simulink model "Gates"  (R2024b)
settings: Solver=FixedStepAuto  StartTime=0  StopTime=1  FixedStep=0.00001  RelTol=1e-3
libraries: spsTriangleGeneratorLib x1
(part 1 of 2)
settings Model: PacingRate=0.110000  Creator=Erys  LastModifiedBy=Erys

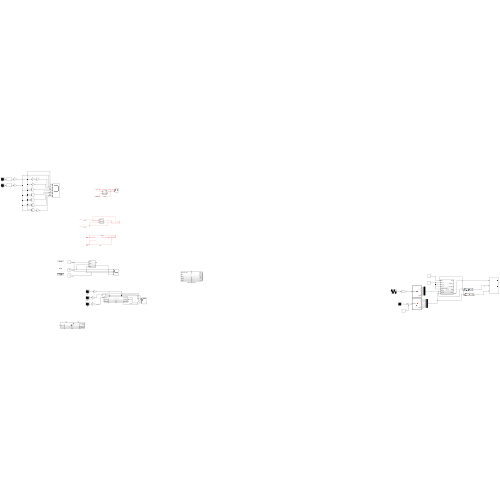
[thumbnail: Simulink's stored preview of the top-level diagram]
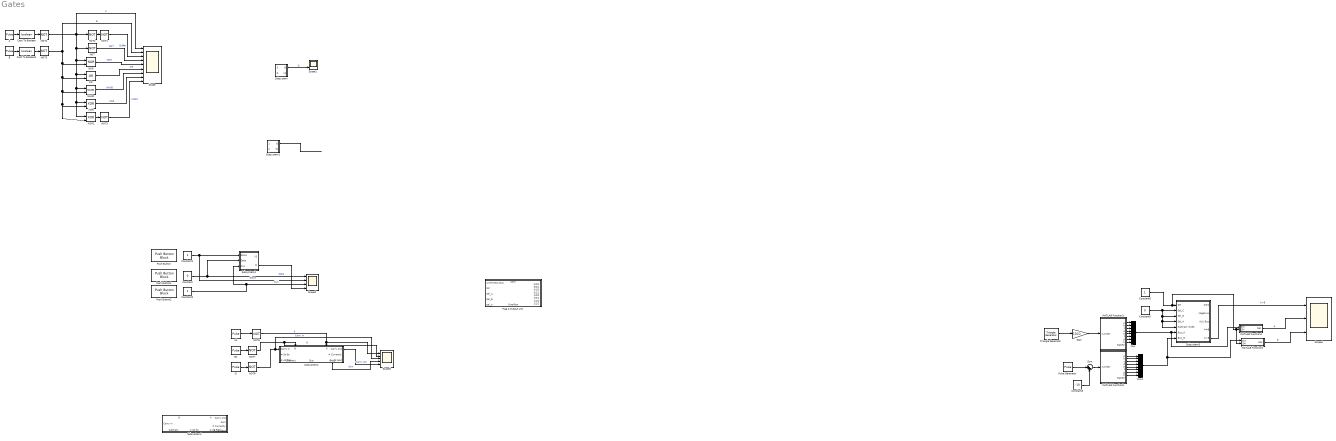
== system Gates ==
  A : DiscretePulseGenerator  PulseType=Time based  Period=1  PulseWidth=50
  A1 : DiscretePulseGenerator  PulseType=Time based  Period=0.25  PulseWidth=50
  B : DiscretePulseGenerator  PulseType=Time based  Period=0.5  PulseWidth=50
  B1 : DiscretePulseGenerator  PulseType=Time based  Period=0.5  PulseWidth=50
  CI : DiscretePulseGenerator  PulseType=Time based  Period=1  PulseWidth=50
  Cast To Boolean : DataTypeConversion  OutDataTypeStr=boolean  SaturateOnIntegerOverflow=off  RndMeth=Floor
  Cast To Boolean1 : DataTypeConversion  OutDataTypeStr=boolean  SaturateOnIntegerOverflow=off  RndMeth=Floor
  Constant : Constant  Value=0  OutDataTypeStr=boolean
  Constant1 : Constant  OutDataTypeStr=boolean
  Constant2 : Constant  OutDataTypeStr=boolean
  Constant3 : Constant  Value=-10
  Constant5 : Constant  Value=0
  Constant6 : Constant
  Flag & Output unit : Subsystem
      settings: PortSchema="{\"entries\":[{\"content\":{\"sides\":[{\"content\":{\"connectorIds\":[\"In1\",\"In2\",\"In3\",\"In4\",\"In5\"]},\"type\":\"ConnectorPlacement.EquallySpacedRectSide\",\"uuid\":\"916d1b19-e284-4a28-84cf-bc055bf0c44e\"},{\"content\":{\"connectorIds\":[\"Out1\",\"Out2\",\"Out3\",\"Out4\",\"Out5\",\"Out6\",\"Out7\",\"Out8\"],\"side\":\"RIGHT\"},\"type\":\"ConnectorPlacement.EquallySpacedRectSide\",\"uuid\":\"7130d779-fd13-4a69-b7b9-2dcd4faf046d\"},{\"content\":{\"connectorIds\":[\"Out9\"],\"side\":\"TOP\"},\"type\":\"ConnectorPlacement.EquallySpacedRectSide\",\"uuid\":\"ce59600e-a31e-4529-9735-bd24f6721c4e\"},{\"content\":{\"connectorIds\":[\"In6\"],\"side\":\"BOTTOM\"},\"type\":\"ConnectorPlacement.EquallySpacedRectSide\",\"uuid\":\"41b3058d-0677-4e1c-be90-f7fc2536099b\"}]},\"type\":\"ConnectorPlacement.EquallySpacedConnector\",\"uuid\":\"b715e1e6-03cb-4b7c-85cc-1984e61b148f\"}],\"packageUris\":[\"http://schema.mathworks.com/mf0/Connector/R2020b\"],\"version\":\"1.0\"}"
  Gain : Gain  Gain=126/2
  MATLAB Function1 : MATLAB Function  TreatAsAtomicUnit=on
  MATLAB Function2 : MATLAB Function  TreatAsAtomicUnit=on
  MATLAB Function3 : MATLAB Function  TreatAsAtomicUnit=on
  MATLAB Function4 : MATLAB Function  TreatAsAtomicUnit=on
  Mux : Mux  Inputs=8
  Mux1 : Mux  Inputs=8
  NAND : Logic  Operator=NAND  IconShape=distinctive  AllPortsSameDT=off  OutDataTypeStr=boolean
  NOR : Logic  Operator=NOR  IconShape=distinctive  AllPortsSameDT=off  OutDataTypeStr=boolean
  NOT{,1..8} (9 alike) : Logic  Operator=NOT  IconShape=distinctive  AllPortsSameDT=off  OutDataTypeStr=boolean
  OR : Logic  Operator=OR  IconShape=distinctive  AllPortsSameDT=off  OutDataTypeStr=boolean
  Pulse Generator : DiscretePulseGenerator  PulseType=Time based  Amplitude=20  Period=1  PulseWidth=50
  Push Button : PushButtonBlock  ButtonType=Latch  OffValue=0.000000
  Push Button1 : PushButtonBlock  ButtonType=Latch  OffValue=0.000000
  Push Button2 : PushButtonBlock  ButtonType=Latch  OffValue=0.000000
  Scope : Scope  NumInputPorts=9
  Scope1 : Scope  NumInputPorts=3
  Scope2 : Scope  NumInputPorts=4
  Scope3 : Scope  NumInputPorts=5
  Scope4 : Scope  NumInputPorts=3
  Subsystem : Subsystem
  Subsystem1 : Subsystem
  Subsystem2 : Subsystem
      settings: PortSchema="{\"entries\":[{\"content\":{\"sides\":[{\"content\":{\"connectorIds\":[\"In1\",\"In2\",\"In3\"]},\"type\":\"ConnectorPlacement.EquallySpacedRectSide\",\"uuid\":\"d566efe6-1fc5-4e96-a6c3-64a47f89d9c9\"},{\"content\":{\"connectorIds\":[\"Out1\",\"Out2\",\"Out3\"],\"side\":\"RIGHT\"},\"type\":\"ConnectorPlacement.EquallySpacedRectSide\",\"uuid\":\"006cd780-973d-4bae-abc8-89f745b28566\"},{\"content\":{\"connectorIds\":[\"In4\",\"In5\"],\"side\":\"TOP\"},\"type\":\"ConnectorPlacement.EquallySpacedRectSide\",\"uuid\":\"c760ecb1-3a5c-4ba0-9224-1c9b5ce710fd\"},{\"content\":{\"connectorIds\":[\"In6\",\"Out4\",\"Out5\"],\"side\":\"BOTTOM\"},\"type\":\"ConnectorPlacement.EquallySpacedRectSide\",\"uuid\":\"178f6c5d-529f-4f0d-80ca-fb6729cf398e\"}]},\"type\":\"ConnectorPlacement.EquallySpacedConnector\",\"uuid\":\"d5293939-72db-46a2-88f3-163e4f70d202\"}],\"packageUris\":[\"http://schema.mathworks.com/mf0/Connector/R2020b\"],\"version\":\"1.0\"}"
  Subsystem3 : Subsystem
  Subsystem4 : Subsystem
      settings: PortSchema="{\"entries\":[{\"content\":{\"sides\":[{\"content\":{\"connectorIds\":[\"In1\"]},\"type\":\"ConnectorPlacement.EquallySpacedRectSide\",\"uuid\":\"d566efe6-1fc5-4e96-a6c3-64a47f89d9c9\"},{\"content\":{\"connectorIds\":[\"Out1\",\"Out2\",\"Out3\",\"Out4\"],\"side\":\"RIGHT\"},\"type\":\"ConnectorPlacement.EquallySpacedRectSide\",\"uuid\":\"006cd780-973d-4bae-abc8-89f745b28566\"},{\"content\":{\"connectorIds\":[\"In2\",\"In3\"],\"side\":\"TOP\"},\"type\":\"ConnectorPlacement.EquallySpacedRectSide\",\"uuid\":\"c760ecb1-3a5c-4ba0-9224-1c9b5ce710fd\"},{\"content\":{\"connectorIds\":[\"In4\",\"In5\",\"In6\"],\"side\":\"BOTTOM\"},\"type\":\"ConnectorPlacement.EquallySpacedRectSide\",\"uuid\":\"178f6c5d-529f-4f0d-80ca-fb6729cf398e\"}]},\"type\":\"ConnectorPlacement.EquallySpacedConnector\",\"uuid\":\"d5293939-72db-46a2-88f3-163e4f70d202\"}],\"packageUris\":[\"http://schema.mathworks.com/mf0/Connector/R2020b\"],\"version\":\"1.0\"}"
  Subsystem5 : Subsystem
  Sum : Sum  Inputs=|++
  Triangle Generator : spsTriangleGeneratorLib/Triangle Generator  Freq=4  Phase=90  Ts=0
  XOR : Logic  Operator=XOR  IconShape=distinctive  AllPortsSameDT=off  OutDataTypeStr=boolean
  XOR1 : Logic  Operator=XOR  IconShape=distinctive  AllPortsSameDT=off  OutDataTypeStr=boolean
  wires:
  NOT2/1 -> NOT1/1
  XOR1/1 -> NOT3/1
  A/1 -> Cast To Boolean/1
  B/1 -> Cast To Boolean1/1
  NOR/1 -> Scope/5  "NOR"
  Cast To Boolean/1 -> NOT4/1
  Cast To Boolean1/1 -> NOT5/1
  NOT4/1 -> XOR1/1, XOR/1, NAND/1, OR/1, NOR/1, NOT/1, Scope/1, NOT2/1  "A"
  NOT5/1 -> XOR1/2, XOR/2, NAND/2, OR/2, NOR/2, Scope/2  "B"
  NOT1/1 -> Scope/3  "Buffer"
  NOT/1 -> Scope/4  "NOT"
  OR/1 -> Scope/6  "OR"
  NAND/1 -> Scope/7  "NAND"
  XOR/1 -> Scope/8  "XOR"
  NOT3/1 -> Scope/9  "XNOR"
  ? -> Scope1/2, Subsystem/2(R)  "Reset"
  ? -> Scope1/1, Subsystem/1(S)  "Set"
  Subsystem/1(Q) -> Scope1/3  "Q"
  ? -> Subsystem1/1(Data)  "Data"
  ? -> Subsystem1/2(CLK)  "CLK"
  Subsystem1/1(Q) -> ?
  ? -> ?  "Data"
  ? -> ?  "CLK"
  ? -> ?  "Q"
  Constant1/1 -> Scope2/2, Subsystem3/1(Store)  "Store"
  Constant/1 -> Scope2/1, Subsystem3/2(Data)  "Data"
  Constant2/1 -> Subsystem3/3(CLK), Scope2/3  "CLK"
  Subsystem3/2(Q) -> Scope2/4
  A1/1 -> NOT6/1
  B1/1 -> NOT7/1
  CI/1 -> NOT8/1
  Subsystem2/5(Out1) -> Scope3/4  "Sum"
  Subsystem2/1(Carry Out) -> Scope3/5  "Carry out"
  NOT6/1 -> Scope3/1, Subsystem2/5(A)  "A"
  NOT7/1 -> Scope3/2, Subsystem2/4(B)  "B"
  NOT8/1 -> Scope3/3, Subsystem2/1(Carry In)  "Carry In"
  MATLAB Function1/8(h) -> Mux/8
  MATLAB Function1/4(d) -> Mux/4
  MATLAB Function1/7(g) -> Mux/7
  MATLAB Function1/6(f) -> Mux/6
  MATLAB Function1/3(c) -> Mux/3
  MATLAB Function1/1(a) -> Mux/1
  MATLAB Function1/5(e) -> Mux/5
  MATLAB Function1/2(b) -> Mux/2
  Constant5/1 -> Subsystem5/5(Subtract mode), Subsystem5/4(Sel_A), Subsystem5/3(Sel_B), Subsystem5/2(Sel_C)
  MATLAB Function3/5(e) -> Mux1/5
  MATLAB Function3/1(a) -> Mux1/1
  MATLAB Function3/2(b) -> Mux1/2
  Mux1/1 -> MATLAB Function2/1(Bin), Subsystem5/7(Bus_B)
  MATLAB Function3/4(d) -> Mux1/4
  MATLAB Function3/7(g) -> Mux1/7
  MATLAB Function3/8(h) -> Mux1/8
  MATLAB Function3/3(c) -> Mux1/3
  MATLAB Function3/6(f) -> Mux1/6
  Mux/1 -> MATLAB Function4/1(Bin), Subsystem5/6(Bus_A)
  MATLAB Function4/1(Dec) -> Scope4/2  "A"
  MATLAB Function2/1(Dec) -> Scope4/3  "B"
  Constant6/1 -> MATLAB Function2/2(SM), MATLAB Function4/2(SM), Subsystem5/1(SM)
  Subsystem5/5(A>B) -> Scope4/1  "A>B"
  Gain/1 -> MATLAB Function1/1(number)
  Triangle Generator/1 -> Gain/1
  Pulse Generator/1 -> Sum/1
  Sum/1 -> MATLAB Function3/1(number)
  Constant3/1 -> Sum/2

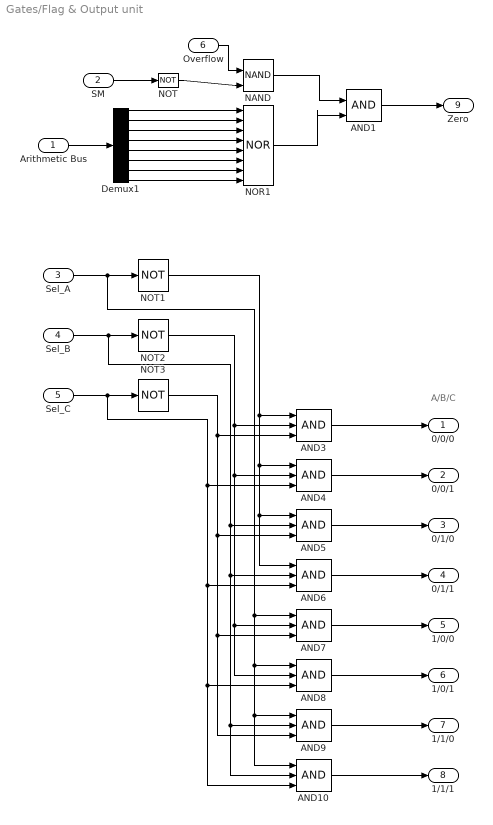
== system Gates/Flag & Output unit ==
  note: A/B/C
  Arithmetic Bus : Inport
  SM : Inport  Port=2
  Sel_A : Inport  Port=3
  Sel_B : Inport  Port=4
  Sel_C : Inport  Port=5
  Overflow : Inport  Port=6
  AND1 : Logic  IconShape=distinctive  AllPortsSameDT=off  OutDataTypeStr=boolean
  AND{3..10} (8 alike) : Logic  Inputs=3  IconShape=distinctive  AllPortsSameDT=off  OutDataTypeStr=boolean
  Demux1 : Demux  Outputs=8
  NAND : Logic  Operator=NAND  IconShape=distinctive  AllPortsSameDT=off  OutDataTypeStr=boolean
  NOR1 : Logic  Operator=NOR  Inputs=8  IconShape=distinctive  AllPortsSameDT=off  OutDataTypeStr=boolean
  NOT{,1..3} (4 alike) : Logic  Operator=NOT  IconShape=distinctive  AllPortsSameDT=off  OutDataTypeStr=boolean
  0/0/0 : Outport
  0/0/1 : Outport  Port=2
  0/1/0 : Outport  Port=3
  0/1/1 : Outport  Port=4
  1/0/0 : Outport  Port=5
  1/0/1 : Outport  Port=6
  1/1/0 : Outport  Port=7
  1/1/1 : Outport  Port=8
  Zero : Outport  Port=9
  wires:
  SM/1 -> NOT/1
  Demux1/1 -> NOR1/1
  NOT/1 -> NAND/2
  Demux1/4 -> NOR1/4
  NOR1/1 -> AND1/2
  Overflow/1 -> NAND/1
  Demux1/5 -> NOR1/5
  NAND/1 -> AND1/1
  Demux1/8 -> NOR1/8
  Demux1/6 -> NOR1/6
  Arithmetic Bus/1 -> Demux1/1
  Demux1/7 -> NOR1/7
  Demux1/3 -> NOR1/3
  AND1/1 -> Zero/1
  Demux1/2 -> NOR1/2
  AND3/1 -> 0/0/0/1
  NOT1/1 -> AND6/1, AND5/1, AND4/1, AND3/1
  AND9/1 -> 1/1/0/1
  Sel_C/1 -> AND10/3, AND8/3, AND6/3, AND4/3, NOT3/1
  AND7/1 -> 1/0/0/1
  AND6/1 -> 0/1/1/1
  NOT2/1 -> AND4/2, AND7/2, AND8/2, AND3/2
  Sel_B/1 -> AND10/2, AND9/2, AND6/2, AND5/2, NOT2/1
  AND4/1 -> 0/0/1/1
  NOT3/1 -> AND9/3, AND7/3, AND5/3, AND3/3
  Sel_A/1 -> AND10/1, AND9/1, AND8/1, AND7/1, NOT1/1
  AND5/1 -> 0/1/0/1
  AND8/1 -> 1/0/1/1
  AND10/1 -> 1/1/1/1

== system Gates/Subsystem ==
  S : Inport
  R : Inport  Port=2
  Delay One Step : Delay  DelayLength=1
  NOR1 : Logic  Operator=NOR  IconShape=distinctive  AllPortsSameDT=off  OutDataTypeStr=boolean
  NOR2 : Logic  Operator=NOR  IconShape=distinctive  AllPortsSameDT=off  OutDataTypeStr=boolean
  Q : Outport
  !Q : Outport  Port=2
  wires:
  Delay One Step/1 -> NOR1/2, Q/1  "Q"
  S/1 -> NOR1/1
  R/1 -> NOR2/2
  NOR1/1 -> !Q/1, NOR2/1
  NOR2/1 -> Delay One Step/1

== system Gates/Subsystem1 ==
  Data : Inport
  CLK : Inport  Port=2
  Delay One Step : Delay  DelayLength=1
  NAND{1..4} (4 alike) : Logic  Operator=NAND  IconShape=distinctive  AllPortsSameDT=off  OutDataTypeStr=boolean
  Q : Outport
  !Q : Outport  Port=2
  wires:
  NAND1/1 -> Delay One Step/1
  NAND4/1 -> NAND2/2
  Delay One Step/1 -> NAND2/1, Q/1  "Q"
  NAND2/1 -> !Q/1, NAND1/2
  NAND3/1 -> NAND4/1, NAND1/1
  CLK/1 -> NAND3/2, NAND4/2
  Data/1 -> NAND3/1

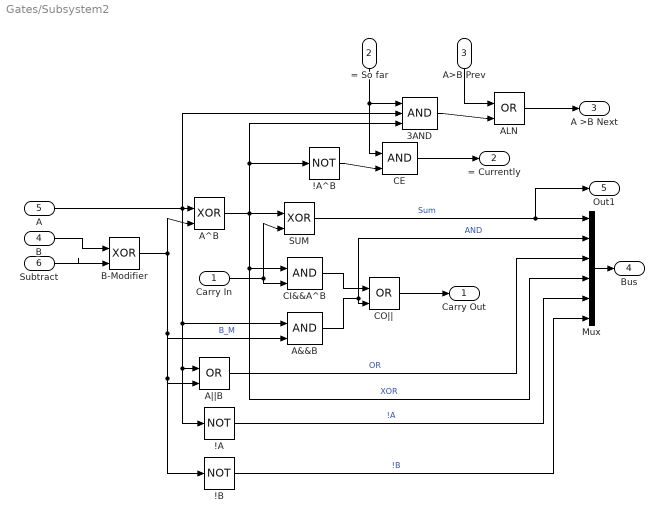
== system Gates/Subsystem2 ==
  Carry In : Inport
  = So far : Inport  Port=2
  A>B Prev : Inport  Port=3
  B : Inport  Port=4
  A : Inport  Port=5
  Subtract : Inport  Port=6
  !A : Logic  Operator=NOT  IconShape=distinctive  AllPortsSameDT=off  OutDataTypeStr=boolean
  !A^B : Logic  Operator=NOT  IconShape=distinctive  AllPortsSameDT=off  OutDataTypeStr=boolean
  !B : Logic  Operator=NOT  IconShape=distinctive  AllPortsSameDT=off  OutDataTypeStr=boolean
  3AND : Logic  Inputs=3  IconShape=distinctive  AllPortsSameDT=off  OutDataTypeStr=boolean
  A&&B : Logic  IconShape=distinctive  AllPortsSameDT=off  OutDataTypeStr=boolean
  ALN : Logic  Operator=OR  IconShape=distinctive  AllPortsSameDT=off  OutDataTypeStr=boolean
  A^B : Logic  Operator=XOR  IconShape=distinctive  AllPortsSameDT=off  OutDataTypeStr=boolean
  A||B : Logic  Operator=OR  IconShape=distinctive  AllPortsSameDT=off  OutDataTypeStr=boolean
  B-Modifier : Logic  Operator=XOR  IconShape=distinctive  AllPortsSameDT=off  OutDataTypeStr=boolean
  CE : Logic  IconShape=distinctive  AllPortsSameDT=off  OutDataTypeStr=boolean
  CI&&A^B : Logic  IconShape=distinctive  AllPortsSameDT=off  OutDataTypeStr=boolean
  CO|| : Logic  Operator=OR  IconShape=distinctive  AllPortsSameDT=off  OutDataTypeStr=boolean
  Mux : Mux  Inputs=6
  SUM : Logic  Operator=XOR  IconShape=distinctive  AllPortsSameDT=off  OutDataTypeStr=boolean
  Carry Out : Outport
  = Currently : Outport  Port=2
  A >B Next : Outport  Port=3
  Bus : Outport  Port=4
  Out1 : Outport  Port=5
  wires:
  B/1 -> B-Modifier/1
  Subtract/1 -> B-Modifier/2
  CI&&A^B/1 -> CO||/1
  A&&B/1 -> Mux/2, CO||/2  "AND"
  CO||/1 -> Carry Out/1
  B-Modifier/1 -> A&&B/2, !B/1, A||B/2, A^B/2  "B_M"
  Carry In/1 -> CI&&A^B/2, SUM/2
  SUM/1 -> Out1/1, Mux/1  "Sum"
  A^B/1 -> Mux/4, CI&&A^B/1, 3AND/3, !A^B/1, SUM/1  "XOR"
  A>B Prev/1 -> ALN/1
  ALN/1 -> A >B Next/1
  !A^B/1 -> CE/2
  CE/1 -> = Currently/1
  3AND/1 -> ALN/2
  A/1 -> !A/1, A||B/1, A&&B/1, A^B/1, 3AND/2
  = So far/1 -> CE/1, 3AND/1
  A||B/1 -> Mux/3  "OR"
  Mux/1 -> Bus/1
  !A/1 -> Mux/5  "!A"
  !B/1 -> Mux/6  "!B"

== system Gates/Subsystem3 ==
  Store : Inport
  Data : Inport  Port=2
  CLK : Inport  Port=3
  NAND1 : Logic  Operator=NAND  IconShape=distinctive  AllPortsSameDT=off  OutDataTypeStr=boolean
  NAND2 : Logic  Operator=NAND  IconShape=distinctive  AllPortsSameDT=off  OutDataTypeStr=boolean
  NAND3 : Logic  Operator=NAND  IconShape=distinctive  AllPortsSameDT=off  OutDataTypeStr=boolean
  NOT6 : Logic  Operator=NOT  IconShape=distinctive  AllPortsSameDT=off  OutDataTypeStr=boolean
  Subsystem2 : Subsystem
  !Q : Outport
  Q : Outport  Port=2
  wires:
  NAND3/1 -> NAND1/2
  Subsystem2/1(Q) -> Q/1, NAND2/1  "Q"
  NAND1/1 -> Subsystem2/1(Data)
  NOT6/1 -> NAND2/2
  CLK/1 -> Subsystem2/2(CLK)
  Store/1 -> NOT6/1, NAND3/1
  NAND2/1 -> NAND1/1
  Subsystem2/2(!Q) -> !Q/1
  Data/1 -> NAND3/2

== system Gates/Subsystem4 ==
  Carry In : Inport
  B : Inport  Port=2
  A : Inport  Port=3
  Subtract : Inport  Port=4
  = So far : Inport  Port=5
  A>B Prev : Inport  Port=6
  !A^B : Logic  Operator=NOT  IconShape=distinctive  AllPortsSameDT=off  OutDataTypeStr=boolean
  AND : Logic  IconShape=distinctive  AllPortsSameDT=off  OutDataTypeStr=boolean
  AND2 : Logic  IconShape=distinctive  AllPortsSameDT=off  OutDataTypeStr=boolean
  AND5 : Logic  IconShape=distinctive  AllPortsSameDT=off  OutDataTypeStr=boolean
  AND6 : Logic  Inputs=3  IconShape=distinctive  AllPortsSameDT=off  OutDataTypeStr=boolean
  OR1 : Logic  Operator=OR  IconShape=distinctive  AllPortsSameDT=off  OutDataTypeStr=boolean
  OR2 : Logic  Operator=OR  IconShape=distinctive  AllPortsSameDT=off  OutDataTypeStr=boolean
  XOR : Logic  Operator=XOR  IconShape=distinctive  AllPortsSameDT=off  OutDataTypeStr=boolean
  XOR1 : Logic  Operator=XOR  IconShape=distinctive  AllPortsSameDT=off  OutDataTypeStr=boolean
  XOR2 : Logic  Operator=XOR  IconShape=distinctive  AllPortsSameDT=off  OutDataTypeStr=boolean
  Carry Out : Outport
  Sum : Outport  Port=2
  = Currently : Outport  Port=3
  A >B Next : Outport  Port=4
  wires:
  B/1 -> XOR1/1
  Subtract/1 -> XOR1/2
  AND/1 -> OR1/1
  AND2/1 -> OR1/2
  OR1/1 -> Carry Out/1
  XOR1/1 -> AND2/2, XOR2/2
  Carry In/1 -> AND/2, XOR/2
  XOR/1 -> Sum/1
  AND5/1 -> = Currently/1
  = So far/1 -> AND6/1, AND5/1
  !A^B/1 -> AND5/2
  XOR2/1 -> AND6/3, !A^B/1, AND/1, XOR/1
  OR2/1 -> A >B Next/1
  A/1 -> AND2/1, AND6/2, XOR2/1
  AND6/1 -> OR2/2
  A>B Prev/1 -> OR2/1

== system Gates/Subsystem5 ==
  SM : Inport
  Sel_C : Inport  Port=2
  Sel_B : Inport  Port=3
  Sel_A : Inport  Port=4
  Subtract mode : Inport  Port=5
  Bus_A : Inport  Port=6
  Bus_B : Inport  Port=7
  ALU Selector Bus : Subsystem
      settings: PortSchema="{\"entries\":[{\"content\":{\"sides\":[{\"content\":{\"connectorIds\":[\"In1\",\"In2\",\"In3\",\"In4\",\"In5\",\"In6\",\"In7\",\"In8\",\"In9\",\"In10\",\"In11\",\"In12\",\"In13\",\"In14\",\"In15\",\"In16\"]},\"type\":\"ConnectorPlacement.EquallySpacedRectSide\",\"uuid\":\"e3413fa4-1b2d-4ebe-83ea-8face2a722c4\"},{\"content\":{\"side\":\"RIGHT\"},\"type\":\"ConnectorPlacement.EquallySpacedRectSide\",\"uuid\":\"468a20b8-3e48-40d2-af84-5907293b05d2\"},{\"content\":{\"connectorIds\":[\"Out1\"],\"side\":\"TOP\"},\"type\":\"ConnectorPlacement.EquallySpacedRectSide\",\"uuid\":\"4c8356f8-7f0f-47fd-8d6e-25cf38d6ddc3\"}]},\"type\":\"ConnectorPlacement.EquallySpacedConnector\",\"uuid\":\"84f87871-f62c-4317-8781-2bab8d5e1233\"}],\"packageUris\":[\"http://schema.mathworks.com/mf0/Connector/R2020b\"],\"version\":\"1.0\"}"
  Adder & Logic Module : Subsystem
      settings: PortSchema="{\"entries\":[{\"content\":{\"sides\":[{\"content\":{\"connectorIds\":[\"In1\",\"In2\"]},\"type\":\"ConnectorPlacement.EquallySpacedRectSide\",\"uuid\":\"639aed8e-35a1-4ba0-8b43-3214fbb2c368\"},{\"content\":{\"connectorIds\":[\"Out1\",\"Out2\",\"Out3\",\"Out4\",\"Out5\",\"Out6\",\"Out7\",\"Out8\"],\"side\":\"RIGHT\"},\"type\":\"ConnectorPlacement.EquallySpacedRectSide\",\"uuid\":\"8a439bfb-ce30-47da-a5b4-a54b9d9e640c\"},{\"content\":{\"connectorIds\":[\"In3\",\"Out11\"],\"side\":\"TOP\"},\"type\":\"ConnectorPlacement.EquallySpacedRectSide\",\"uuid\":\"7d81641d-429b-4b81-8cb3-af5c318085c9\"},{\"content\":{\"connectorIds\":[\"Out9\",\"Out10\"],\"side\":\"BOTTOM\"},\"type\":\"ConnectorPlacement.EquallySpacedRectSide\",\"uuid\":\"74152c7b-6851-457b-b5de-2c09c1f82f74\"}]},\"type\":\"ConnectorPlacement.EquallySpacedConnector\",\"uuid\":\"d9b5c2cc-0f19-487b-a2d0-c7259543056d\"}],\"packageUris\":[\"http://schema.mathworks.com/mf0/Connector/R2020b\"],\"version\":\"1.0\"}"
  Flag & Output unit1 : Subsystem
      settings: PortSchema="{\"entries\":[{\"content\":{\"sides\":[{\"content\":{\"connectorIds\":[\"In1\",\"In2\",\"In3\",\"In4\"]},\"type\":\"ConnectorPlacement.EquallySpacedRectSide\",\"uuid\":\"916d1b19-e284-4a28-84cf-bc055bf0c44e\"},{\"content\":{\"connectorIds\":[\"Out1\",\"Out2\",\"Out3\",\"Out4\",\"Out5\",\"Out6\",\"Out7\",\"Out8\"],\"side\":\"RIGHT\"},\"type\":\"ConnectorPlacement.EquallySpacedRectSide\",\"uuid\":\"7130d779-fd13-4a69-b7b9-2dcd4faf046d\"},{\"content\":{\"connectorIds\":[\"Out9\",\"Out10\",\"In5\"],\"side\":\"TOP\"},\"type\":\"ConnectorPlacement.EquallySpacedRectSide\",\"uuid\":\"ce59600e-a31e-4529-9735-bd24f6721c4e\"},{\"content\":{\"connectorIds\":[\"In6\"],\"side\":\"BOTTOM\"},\"type\":\"ConnectorPlacement.EquallySpacedRectSide\",\"uuid\":\"41b3058d-0677-4e1c-be90-f7fc2536099b\"}]},\"type\":\"ConnectorPlacement.EquallySpacedConnector\",\"uuid\":\"b715e1e6-03cb-4b7c-85cc-1984e61b148f\"}],\"packageUris\":[\"http://schema.mathworks.com/mf0/Connector/R2020b\"],\"version\":\"1.0\"}"
  Zero : Outport
  Negative : Outport  Port=2
  ALU Bus : Outport  Port=3
  A=B : Outport  Port=4
  A>B : Outport  Port=5
  wires:
  Subtract mode/1 -> Adder & Logic Module/3(Subtract mode)
  Bus_B/1 -> Adder & Logic Module/2(Bus_B)
  Bus_A/1 -> Adder & Logic Module/1(Bus_A)
  Adder & Logic Module/10(A>B) -> A>B/1
  Adder & Logic Module/7(Bus7) -> ALU Selector Bus/15(Bus7)
  Adder & Logic Module/5(Bus5) -> ALU Selector Bus/13(Bus5)
  Adder & Logic Module/3(Bus3) -> ALU Selector Bus/11(Bus3)
  Adder & Logic Module/9(A=B) -> A=B/1
  SM/1 -> Flag & Output unit1/1(SM)
  Sel_B/1 -> Flag & Output unit1/3(Sel_B)
  Sel_A/1 -> Flag & Output unit1/2(Sel_A)
  Sel_C/1 -> Flag & Output unit1/4(Sel_C)
  Adder & Logic Module/1(Bus1) -> ALU Selector Bus/9(Bus1)
  Adder & Logic Module/8(Bus8) -> ALU Selector Bus/16(Bus8)
  Adder & Logic Module/6(Bus6) -> ALU Selector Bus/14(Bus6)
  Adder & Logic Module/4(Bus4) -> ALU Selector Bus/12(Bus4)
  Adder & Logic Module/2(Bus2) -> ALU Selector Bus/10(Bus2)
  Adder & Logic Module/11(Overflow) -> Flag & Output unit1/6(Overflow)
  Flag & Output unit1/5(1/0/0) -> ALU Selector Bus/5(1/0/0)
  Flag & Output unit1/3(0/1/0) -> ALU Selector Bus/3(0/1/0)
  Flag & Output unit1/1(0/0/0) -> ALU Selector Bus/1(0/0/0)
  Flag & Output unit1/4(0/1/1) -> ALU Selector Bus/4(0/1/1)
  Flag & Output unit1/2(0/0/1) -> ALU Selector Bus/2(0/0/1)
  Flag & Output unit1/10(Negative) -> Negative/1
  Flag & Output unit1/8(1/1/1) -> ALU Selector Bus/8(1/1/1)
  Flag & Output unit1/6(1/0/1) -> ALU Selector Bus/6(1/0/1)
  Flag & Output unit1/9(Zero) -> Zero/1
  Flag & Output unit1/7(1/1/0) -> ALU Selector Bus/7(1/1/0)
  ALU Selector Bus/1(ALU Output) -> Flag & Output unit1/5(ALU Bus), ALU Bus/1

== system Gates/Subsystem3/Subsystem2 ==
  Data : Inport
  CLK : Inport  Port=2
  DLatch Master : Subsystem
  DLatch Slave : Subsystem
  NOT6 : Logic  Operator=NOT  IconShape=distinctive  AllPortsSameDT=off  OutDataTypeStr=boolean
  Q : Outport
  !Q : Outport  Port=2
  wires:
  DLatch Master/1(Q) -> DLatch Slave/1(Data)
  NOT6/1 -> DLatch Master/2(CLK)
  CLK/1 -> DLatch Slave/2(CLK), NOT6/1
  Data/1 -> DLatch Master/1(Data)
  DLatch Slave/1(Q) -> Q/1
  DLatch Slave/2(!Q) -> !Q/1

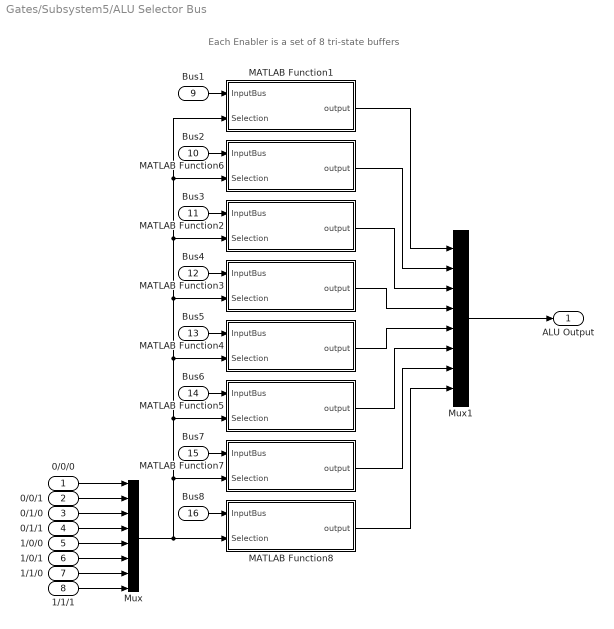
== system Gates/Subsystem5/ALU Selector Bus ==
  note: Each Enabler is a set of 8 tri-state buffers
  0/0/0 : Inport
  0/0/1 : Inport  Port=2
  0/1/0 : Inport  Port=3
  0/1/1 : Inport  Port=4
  1/0/0 : Inport  Port=5
  1/0/1 : Inport  Port=6
  1/1/0 : Inport  Port=7
  1/1/1 : Inport  Port=8
  Bus1 : Inport  Port=9
  Bus2 : Inport  Port=10
  Bus3 : Inport  Port=11
  Bus4 : Inport  Port=12
  Bus5 : Inport  Port=13
  Bus6 : Inport  Port=14
  Bus7 : Inport  Port=15
  Bus8 : Inport  Port=16
  MATLAB Function1 : MATLAB Function  TreatAsAtomicUnit=on
  MATLAB Function2 : MATLAB Function  TreatAsAtomicUnit=on
  MATLAB Function3 : MATLAB Function  TreatAsAtomicUnit=on
  MATLAB Function4 : MATLAB Function  TreatAsAtomicUnit=on
  MATLAB Function5 : MATLAB Function  TreatAsAtomicUnit=on
  MATLAB Function6 : MATLAB Function  TreatAsAtomicUnit=on
  MATLAB Function7 : MATLAB Function  TreatAsAtomicUnit=on
  MATLAB Function8 : MATLAB Function  TreatAsAtomicUnit=on
  Mux : Mux  Inputs=8
  Mux1 : Mux  Inputs=8
  ALU Output : Outport
  wires:
  1/1/1/1 -> Mux/8
  1/1/0/1 -> Mux/7
  1/0/1/1 -> Mux/6
  1/0/0/1 -> Mux/5
  0/1/1/1 -> Mux/4
  0/1/0/1 -> Mux/3
  0/0/1/1 -> Mux/2
  0/0/0/1 -> Mux/1
  Bus3/1 -> MATLAB Function2/1(InputBus)
  Bus5/1 -> MATLAB Function4/1(InputBus)
  Bus8/1 -> MATLAB Function8/1(InputBus)
  Bus2/1 -> MATLAB Function6/1(InputBus)
  Bus4/1 -> MATLAB Function3/1(InputBus)
  Bus1/1 -> MATLAB Function1/1(InputBus)
  Bus6/1 -> MATLAB Function5/1(InputBus)
  Bus7/1 -> MATLAB Function7/1(InputBus)
  Mux/1 -> MATLAB Function8/2(Selection), MATLAB Function7/2(Selection), MATLAB Function5/2(Selection), MATLAB Function4/2(Selection), MATLAB Function3/2(Selection), MATLAB Function2/2(Selection), MATLAB Function1/2(Selection), MATLAB Function6/2(Selection)
  MATLAB Function6/1(output) -> Mux1/2
  MATLAB Function2/1(output) -> Mux1/3
  MATLAB Function3/1(output) -> Mux1/4
  MATLAB Function4/1(output) -> Mux1/5
  MATLAB Function5/1(output) -> Mux1/6
  MATLAB Function7/1(output) -> Mux1/7
  MATLAB Function8/1(output) -> Mux1/8
  MATLAB Function1/1(output) -> Mux1/1
  Mux1/1 -> ALU Output/1

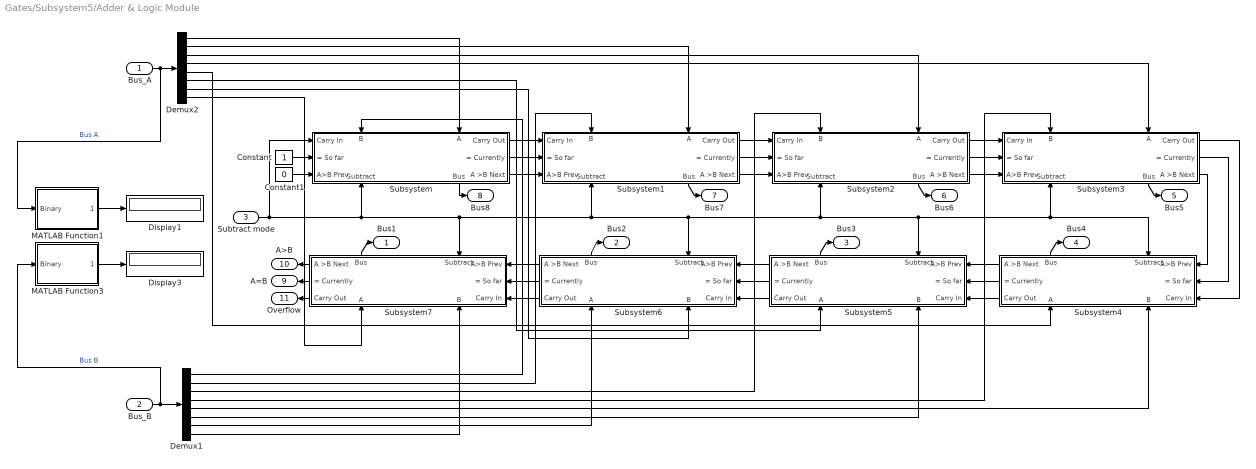
== system Gates/Subsystem5/Adder & Logic Module ==
  Bus_A : Inport
  Bus_B : Inport  Port=2
  Subtract mode : Inport  Port=3
  Constant : Constant
  Constant1 : Constant  Value=0
  Demux1 : Demux  Outputs=8
  Demux2 : Demux  Outputs=8
  Display1 : Display
  Display3 : Display
  MATLAB Function1 : MATLAB Function  TreatAsAtomicUnit=on
  MATLAB Function3 : MATLAB Function  TreatAsAtomicUnit=on
  Subsystem : Subsystem
      settings: PortSchema="{\"entries\":[{\"content\":{\"sides\":[{\"content\":{\"connectorIds\":[\"In1\",\"In2\",\"In3\"]},\"type\":\"ConnectorPlacement.EquallySpacedRectSide\",\"uuid\":\"d566efe6-1fc5-4e96-a6c3-64a47f89d9c9\"},{\"content\":{\"connectorIds\":[\"Out1\",\"Out2\",\"Out3\"],\"side\":\"RIGHT\"},\"type\":\"ConnectorPlacement.EquallySpacedRectSide\",\"uuid\":\"006cd780-973d-4bae-abc8-89f745b28566\"},{\"content\":{\"connectorIds\":[\"In4\",\"In5\"],\"side\":\"TOP\"},\"type\":\"ConnectorPlacement.EquallySpacedRectSide\",\"uuid\":\"c760ecb1-3a5c-4ba0-9224-1c9b5ce710fd\"},{\"content\":{\"connectorIds\":[\"In6\",\"Out4\"],\"side\":\"BOTTOM\"},\"type\":\"ConnectorPlacement.EquallySpacedRectSide\",\"uuid\":\"178f6c5d-529f-4f0d-80ca-fb6729cf398e\"}]},\"type\":\"ConnectorPlacement.EquallySpacedConnector\",\"uuid\":\"d5293939-72db-46a2-88f3-163e4f70d202\"}],\"packageUris\":[\"http://schema.mathworks.com/mf0/Connector/R2020b\"],\"version\":\"1.0\"}"
  Subsystem1 : Subsystem
      settings: PortSchema="{\"entries\":[{\"content\":{\"sides\":[{\"content\":{\"connectorIds\":[\"In1\",\"In2\",\"In3\"]},\"type\":\"ConnectorPlacement.EquallySpacedRectSide\",\"uuid\":\"d566efe6-1fc5-4e96-a6c3-64a47f89d9c9\"},{\"content\":{\"connectorIds\":[\"Out1\",\"Out2\",\"Out3\"],\"side\":\"RIGHT\"},\"type\":\"ConnectorPlacement.EquallySpacedRectSide\",\"uuid\":\"006cd780-973d-4bae-abc8-89f745b28566\"},{\"content\":{\"connectorIds\":[\"In4\",\"In5\"],\"side\":\"TOP\"},\"type\":\"ConnectorPlacement.EquallySpacedRectSide\",\"uuid\":\"c760ecb1-3a5c-4ba0-9224-1c9b5ce710fd\"},{\"content\":{\"connectorIds\":[\"In6\",\"Out4\"],\"side\":\"BOTTOM\"},\"type\":\"ConnectorPlacement.EquallySpacedRectSide\",\"uuid\":\"178f6c5d-529f-4f0d-80ca-fb6729cf398e\"}]},\"type\":\"ConnectorPlacement.EquallySpacedConnector\",\"uuid\":\"d5293939-72db-46a2-88f3-163e4f70d202\"}],\"packageUris\":[\"http://schema.mathworks.com/mf0/Connector/R2020b\"],\"version\":\"1.0\"}"
  Subsystem2 : Subsystem
      settings: PortSchema="{\"entries\":[{\"content\":{\"sides\":[{\"content\":{\"connectorIds\":[\"In1\",\"In2\",\"In3\"]},\"type\":\"ConnectorPlacement.EquallySpacedRectSide\",\"uuid\":\"d566efe6-1fc5-4e96-a6c3-64a47f89d9c9\"},{\"content\":{\"connectorIds\":[\"Out1\",\"Out2\",\"Out3\"],\"side\":\"RIGHT\"},\"type\":\"ConnectorPlacement.EquallySpacedRectSide\",\"uuid\":\"006cd780-973d-4bae-abc8-89f745b28566\"},{\"content\":{\"connectorIds\":[\"In4\",\"In5\"],\"side\":\"TOP\"},\"type\":\"ConnectorPlacement.EquallySpacedRectSide\",\"uuid\":\"c760ecb1-3a5c-4ba0-9224-1c9b5ce710fd\"},{\"content\":{\"connectorIds\":[\"In6\",\"Out4\"],\"side\":\"BOTTOM\"},\"type\":\"ConnectorPlacement.EquallySpacedRectSide\",\"uuid\":\"178f6c5d-529f-4f0d-80ca-fb6729cf398e\"}]},\"type\":\"ConnectorPlacement.EquallySpacedConnector\",\"uuid\":\"d5293939-72db-46a2-88f3-163e4f70d202\"}],\"packageUris\":[\"http://schema.mathworks.com/mf0/Connector/R2020b\"],\"version\":\"1.0\"}"
  Subsystem3 : Subsystem
      settings: PortSchema="{\"entries\":[{\"content\":{\"sides\":[{\"content\":{\"connectorIds\":[\"In1\",\"In2\",\"In3\"]},\"type\":\"ConnectorPlacement.EquallySpacedRectSide\",\"uuid\":\"d566efe6-1fc5-4e96-a6c3-64a47f89d9c9\"},{\"content\":{\"connectorIds\":[\"Out1\",\"Out2\",\"Out3\"],\"side\":\"RIGHT\"},\"type\":\"ConnectorPlacement.EquallySpacedRectSide\",\"uuid\":\"006cd780-973d-4bae-abc8-89f745b28566\"},{\"content\":{\"connectorIds\":[\"In4\",\"In5\"],\"side\":\"TOP\"},\"type\":\"ConnectorPlacement.EquallySpacedRectSide\",\"uuid\":\"c760ecb1-3a5c-4ba0-9224-1c9b5ce710fd\"},{\"content\":{\"connectorIds\":[\"In6\",\"Out4\"],\"side\":\"BOTTOM\"},\"type\":\"ConnectorPlacement.EquallySpacedRectSide\",\"uuid\":\"178f6c5d-529f-4f0d-80ca-fb6729cf398e\"}]},\"type\":\"ConnectorPlacement.EquallySpacedConnector\",\"uuid\":\"d5293939-72db-46a2-88f3-163e4f70d202\"}],\"packageUris\":[\"http://schema.mathworks.com/mf0/Connector/R2020b\"],\"version\":\"1.0\"}"
  Subsystem4 : Subsystem
      settings: PortSchema="{\"entries\":[{\"content\":{\"sides\":[{\"content\":{\"connectorIds\":[\"In1\",\"In2\",\"In3\"]},\"type\":\"ConnectorPlacement.EquallySpacedRectSide\",\"uuid\":\"d566efe6-1fc5-4e96-a6c3-64a47f89d9c9\"},{\"content\":{\"connectorIds\":[\"Out1\",\"Out2\",\"Out3\"],\"side\":\"RIGHT\"},\"type\":\"ConnectorPlacement.EquallySpacedRectSide\",\"uuid\":\"006cd780-973d-4bae-abc8-89f745b28566\"},{\"content\":{\"connectorIds\":[\"In4\",\"In5\"],\"side\":\"TOP\"},\"type\":\"ConnectorPlacement.EquallySpacedRectSide\",\"uuid\":\"c760ecb1-3a5c-4ba0-9224-1c9b5ce710fd\"},{\"content\":{\"connectorIds\":[\"In6\",\"Out4\"],\"side\":\"BOTTOM\"},\"type\":\"ConnectorPlacement.EquallySpacedRectSide\",\"uuid\":\"178f6c5d-529f-4f0d-80ca-fb6729cf398e\"}]},\"type\":\"ConnectorPlacement.EquallySpacedConnector\",\"uuid\":\"d5293939-72db-46a2-88f3-163e4f70d202\"}],\"packageUris\":[\"http://schema.mathworks.com/mf0/Connector/R2020b\"],\"version\":\"1.0\"}"
  Subsystem5 : Subsystem
      settings: PortSchema="{\"entries\":[{\"content\":{\"sides\":[{\"content\":{\"connectorIds\":[\"In1\",\"In2\",\"In3\"]},\"type\":\"ConnectorPlacement.EquallySpacedRectSide\",\"uuid\":\"d566efe6-1fc5-4e96-a6c3-64a47f89d9c9\"},{\"content\":{\"connectorIds\":[\"Out1\",\"Out2\",\"Out3\"],\"side\":\"RIGHT\"},\"type\":\"ConnectorPlacement.EquallySpacedRectSide\",\"uuid\":\"006cd780-973d-4bae-abc8-89f745b28566\"},{\"content\":{\"connectorIds\":[\"In4\",\"In5\"],\"side\":\"TOP\"},\"type\":\"ConnectorPlacement.EquallySpacedRectSide\",\"uuid\":\"c760ecb1-3a5c-4ba0-9224-1c9b5ce710fd\"},{\"content\":{\"connectorIds\":[\"In6\",\"Out4\"],\"side\":\"BOTTOM\"},\"type\":\"ConnectorPlacement.EquallySpacedRectSide\",\"uuid\":\"178f6c5d-529f-4f0d-80ca-fb6729cf398e\"}]},\"type\":\"ConnectorPlacement.EquallySpacedConnector\",\"uuid\":\"d5293939-72db-46a2-88f3-163e4f70d202\"}],\"packageUris\":[\"http://schema.mathworks.com/mf0/Connector/R2020b\"],\"version\":\"1.0\"}"
  Subsystem6 : Subsystem
      settings: PortSchema="{\"entries\":[{\"content\":{\"sides\":[{\"content\":{\"connectorIds\":[\"In1\",\"In2\",\"In3\"]},\"type\":\"ConnectorPlacement.EquallySpacedRectSide\",\"uuid\":\"d566efe6-1fc5-4e96-a6c3-64a47f89d9c9\"},{\"content\":{\"connectorIds\":[\"Out1\",\"Out2\",\"Out3\"],\"side\":\"RIGHT\"},\"type\":\"ConnectorPlacement.EquallySpacedRectSide\",\"uuid\":\"006cd780-973d-4bae-abc8-89f745b28566\"},{\"content\":{\"connectorIds\":[\"In4\",\"In5\"],\"side\":\"TOP\"},\"type\":\"ConnectorPlacement.EquallySpacedRectSide\",\"uuid\":\"c760ecb1-3a5c-4ba0-9224-1c9b5ce710fd\"},{\"content\":{\"connectorIds\":[\"In6\",\"Out4\"],\"side\":\"BOTTOM\"},\"type\":\"ConnectorPlacement.EquallySpacedRectSide\",\"uuid\":\"178f6c5d-529f-4f0d-80ca-fb6729cf398e\"}]},\"type\":\"ConnectorPlacement.EquallySpacedConnector\",\"uuid\":\"d5293939-72db-46a2-88f3-163e4f70d202\"}],\"packageUris\":[\"http://schema.mathworks.com/mf0/Connector/R2020b\"],\"version\":\"1.0\"}"
  Subsystem7 : Subsystem
      settings: PortSchema="{\"entries\":[{\"content\":{\"sides\":[{\"content\":{\"connectorIds\":[\"In1\",\"In2\",\"In3\"]},\"type\":\"ConnectorPlacement.EquallySpacedRectSide\",\"uuid\":\"d566efe6-1fc5-4e96-a6c3-64a47f89d9c9\"},{\"content\":{\"connectorIds\":[\"Out1\",\"Out2\",\"Out3\"],\"side\":\"RIGHT\"},\"type\":\"ConnectorPlacement.EquallySpacedRectSide\",\"uuid\":\"006cd780-973d-4bae-abc8-89f745b28566\"},{\"content\":{\"connectorIds\":[\"In4\",\"In5\"],\"side\":\"TOP\"},\"type\":\"ConnectorPlacement.EquallySpacedRectSide\",\"uuid\":\"c760ecb1-3a5c-4ba0-9224-1c9b5ce710fd\"},{\"content\":{\"connectorIds\":[\"In6\",\"Out4\"],\"side\":\"BOTTOM\"},\"type\":\"ConnectorPlacement.EquallySpacedRectSide\",\"uuid\":\"178f6c5d-529f-4f0d-80ca-fb6729cf398e\"}]},\"type\":\"ConnectorPlacement.EquallySpacedConnector\",\"uuid\":\"d5293939-72db-46a2-88f3-163e4f70d202\"}],\"packageUris\":[\"http://schema.mathworks.com/mf0/Connector/R2020b\"],\"version\":\"1.0\"}"
  Bus1 : Outport
  Bus2 : Outport  Port=2
  Bus3 : Outport  Port=3
  Bus4 : Outport  Port=4
  Bus5 : Outport  Port=5
  Bus6 : Outport  Port=6
  Bus7 : Outport  Port=7
  Bus8 : Outport  Port=8
  A=B : Outport  Port=9
  A>B : Outport  Port=10
  Overflow : Outport  Port=11
  wires:
  Subsystem/1(Carry Out) -> Subsystem1/1(Carry In)
  Subsystem/2(= Currently) -> Subsystem1/2(= So far)
  Subsystem/3(A >B Next) -> Subsystem1/3(A>B Prev)
  Subsystem1/2(= Currently) -> Subsystem2/2(= So far)
  Subsystem1/1(Carry Out) -> Subsystem2/1(Carry In)
  Subsystem1/3(A >B Next) -> Subsystem2/3(A>B Prev)
  Subsystem2/2(= Currently) -> Subsystem3/2(= So far)
  Subsystem2/3(A >B Next) -> Subsystem3/3(A>B Prev)
  Subsystem2/1(Carry Out) -> Subsystem3/1(Carry In)
  Subsystem6/2(= Currently) -> Subsystem7/2(= So far)
  Subsystem6/3(A >B Next) -> Subsystem7/3(A>B Prev)
  Subsystem6/1(Carry Out) -> Subsystem7/1(Carry In)
  Subsystem4/2(= Currently) -> Subsystem5/2(= So far)
  Subsystem4/1(Carry Out) -> Subsystem5/1(Carry In)
  Subsystem4/3(A >B Next) -> Subsystem5/3(A>B Prev)
  Subsystem5/2(= Currently) -> Subsystem6/2(= So far)
  Subsystem5/3(A >B Next) -> Subsystem6/3(A>B Prev)
  Subsystem5/1(Carry Out) -> Subsystem6/1(Carry In)
  Subsystem3/3(A >B Next) -> Subsystem4/3(A>B Prev)
  Subsystem3/2(= Currently) -> Subsystem4/2(= So far)
  Subsystem3/1(Carry Out) -> Subsystem4/1(Carry In)
  Subsystem/4(Bus) -> Bus8/1
  Subsystem7/4(Bus) -> Bus1/1
  Subsystem6/4(Bus) -> Bus2/1
  Subsystem5/4(Bus) -> Bus3/1
  Subsystem4/4(Bus) -> Bus4/1
  Subsystem3/4(Bus) -> Bus5/1
  Subsystem2/4(Bus) -> Bus6/1
  Subsystem1/4(Bus) -> Bus7/1
  Subtract mode/1 -> Subsystem/6(Subtract), Subsystem1/6(Subtract), Subsystem6/6(Subtract), Subsystem2/6(Subtract), Subsystem3/6(Subtract), Subsystem4/6(Subtract), Subsystem5/6(Subtract), Subsystem7/6(Subtract), Subsystem/1(Carry In)
  Constant/1 -> Subsystem/2(= So far)
  Constant1/1 -> Subsystem/3(A>B Prev)
  Subsystem7/3(A >B Next) -> A>B/1
  Subsystem7/2(= Currently) -> A=B/1
  Subsystem7/1(Carry Out) -> Overflow/1
  Bus_A/1 -> MATLAB Function1/1(Binary), Demux2/1  "Bus A"
  MATLAB Function1/1(Decimal) -> Display1/1
  Bus_B/1 -> MATLAB Function3/1(Binary), Demux1/1  "Bus B"
  MATLAB Function3/1(Decimal) -> Display3/1
  Demux2/1 -> Subsystem/5(A)
  Demux2/2 -> Subsystem1/5(A)
  Demux2/3 -> Subsystem2/5(A)
  Demux2/4 -> Subsystem3/5(A)
  Demux2/5 -> Subsystem4/5(A)
  Demux2/8 -> Subsystem7/5(A)
  Demux2/7 -> Subsystem6/4(B)
  Demux2/6 -> Subsystem5/5(A)
  Demux1/1 -> Subsystem/4(B)
  Demux1/2 -> Subsystem1/4(B)
  Demux1/3 -> Subsystem2/4(B)
  Demux1/5 -> Subsystem4/4(B)
  Demux1/4 -> Subsystem3/4(B)
  Demux1/6 -> Subsystem5/4(B)
  Demux1/7 -> Subsystem6/5(A)
  Demux1/8 -> Subsystem7/4(B)

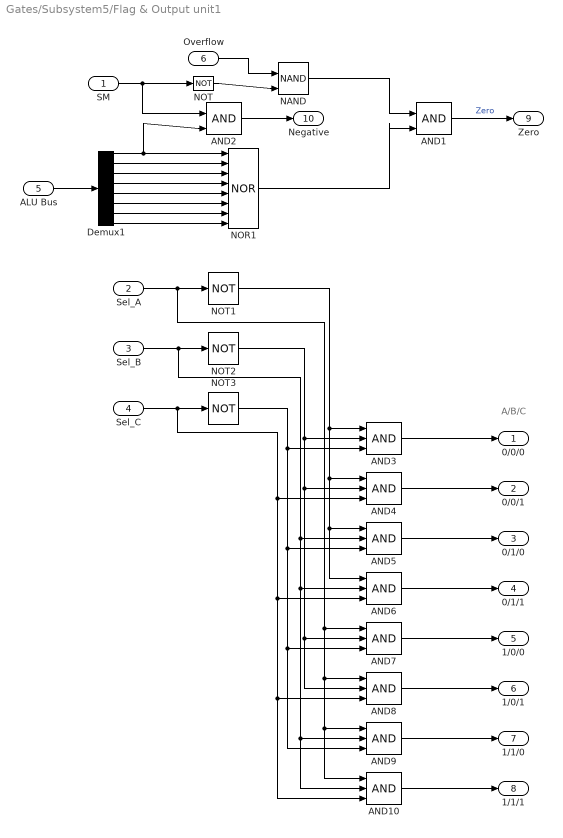
== system Gates/Subsystem5/Flag & Output unit1 ==
  note: A/B/C
  SM : Inport
  Sel_A : Inport  Port=2
  Sel_B : Inport  Port=3
  Sel_C : Inport  Port=4
  ALU Bus : Inport  Port=5
  Overflow : Inport  Port=6
  AND1 : Logic  IconShape=distinctive  AllPortsSameDT=off  OutDataTypeStr=boolean
  AND{3..10} (8 alike) : Logic  Inputs=3  IconShape=distinctive  AllPortsSameDT=off  OutDataTypeStr=boolean
  AND2 : Logic  IconShape=distinctive  AllPortsSameDT=off  OutDataTypeStr=boolean
  Demux1 : Demux  Outputs=8
  NAND : Logic  Operator=NAND  IconShape=distinctive  AllPortsSameDT=off  OutDataTypeStr=boolean
  NOR1 : Logic  Operator=NOR  Inputs=8  IconShape=distinctive  AllPortsSameDT=off  OutDataTypeStr=boolean
  NOT{,1..3} (4 alike) : Logic  Operator=NOT  IconShape=distinctive  AllPortsSameDT=off  OutDataTypeStr=boolean
  0/0/0 : Outport
  0/0/1 : Outport  Port=2
  0/1/0 : Outport  Port=3
  0/1/1 : Outport  Port=4
  1/0/0 : Outport  Port=5
  1/0/1 : Outport  Port=6
  1/1/0 : Outport  Port=7
  1/1/1 : Outport  Port=8
  Zero : Outport  Port=9
  Negative : Outport  Port=10
  wires:
  SM/1 -> AND2/1, NOT/1
  Demux1/1 -> NOR1/1, AND2/2
  NOT/1 -> NAND/2
  Demux1/4 -> NOR1/4
  NOR1/1 -> AND1/2
  Overflow/1 -> NAND/1
  Demux1/5 -> NOR1/5
  NAND/1 -> AND1/1
  Demux1/8 -> NOR1/8
  Demux1/6 -> NOR1/6
  ALU Bus/1 -> Demux1/1
  Demux1/7 -> NOR1/7
  Demux1/3 -> NOR1/3
  AND1/1 -> Zero/1  "Zero"
  AND2/1 -> Negative/1
  Demux1/2 -> NOR1/2
  AND3/1 -> 0/0/0/1
  NOT1/1 -> AND6/1, AND5/1, AND4/1, AND3/1
  AND9/1 -> 1/1/0/1
  Sel_C/1 -> AND10/3, AND8/3, AND6/3, AND4/3, NOT3/1
  AND7/1 -> 1/0/0/1
  AND6/1 -> 0/1/1/1
  NOT2/1 -> AND4/2, AND7/2, AND8/2, AND3/2
  Sel_B/1 -> AND10/2, AND9/2, AND6/2, AND5/2, NOT2/1
  AND4/1 -> 0/0/1/1
  NOT3/1 -> AND9/3, AND7/3, AND5/3, AND3/3
  Sel_A/1 -> AND10/1, AND9/1, AND8/1, AND7/1, NOT1/1
  AND5/1 -> 0/1/0/1
  AND8/1 -> 1/0/1/1
  AND10/1 -> 1/1/1/1

== system Gates/Subsystem3/Subsystem2/DLatch Master ==
  Data : Inport
  CLK : Inport  Port=2
  Delay One Step : Delay  DelayLength=1
  NAND{1..4} (4 alike) : Logic  Operator=NAND  IconShape=distinctive  AllPortsSameDT=off  OutDataTypeStr=boolean
  Q : Outport
  !Q : Outport  Port=2
  wires:
  NAND1/1 -> Delay One Step/1
  NAND4/1 -> NAND2/2
  Delay One Step/1 -> NAND2/1, Q/1  "Q"
  NAND2/1 -> !Q/1, NAND1/2
  NAND3/1 -> NAND4/1, NAND1/1
  CLK/1 -> NAND3/2, NAND4/2
  Data/1 -> NAND3/1

== system Gates/Subsystem3/Subsystem2/DLatch Slave ==
  Data : Inport
  CLK : Inport  Port=2
  Delay One Step : Delay  DelayLength=1
  NAND{1..4} (4 alike) : Logic  Operator=NAND  IconShape=distinctive  AllPortsSameDT=off  OutDataTypeStr=boolean
  Q : Outport
  !Q : Outport  Port=2
  wires:
  NAND1/1 -> Delay One Step/1
  NAND4/1 -> NAND2/2
  Delay One Step/1 -> NAND2/1, Q/1  "Q"
  NAND2/1 -> !Q/1, NAND1/2
  NAND3/1 -> NAND4/1, NAND1/1
  CLK/1 -> NAND3/2, NAND4/2
  Data/1 -> NAND3/1

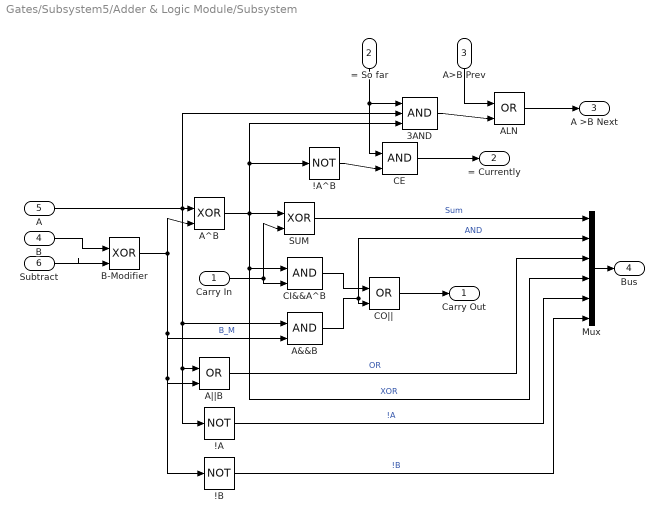
== system Gates/Subsystem5/Adder & Logic Module/Subsystem ==
  Carry In : Inport
  = So far : Inport  Port=2
  A>B Prev : Inport  Port=3
  B : Inport  Port=4
  A : Inport  Port=5
  Subtract : Inport  Port=6
  !A : Logic  Operator=NOT  IconShape=distinctive  AllPortsSameDT=off  OutDataTypeStr=boolean
  !A^B : Logic  Operator=NOT  IconShape=distinctive  AllPortsSameDT=off  OutDataTypeStr=boolean
  !B : Logic  Operator=NOT  IconShape=distinctive  AllPortsSameDT=off  OutDataTypeStr=boolean
  3AND : Logic  Inputs=3  IconShape=distinctive  AllPortsSameDT=off  OutDataTypeStr=boolean
  A&&B : Logic  IconShape=distinctive  AllPortsSameDT=off  OutDataTypeStr=boolean
  ALN : Logic  Operator=OR  IconShape=distinctive  AllPortsSameDT=off  OutDataTypeStr=boolean
  A^B : Logic  Operator=XOR  IconShape=distinctive  AllPortsSameDT=off  OutDataTypeStr=boolean
  A||B : Logic  Operator=OR  IconShape=distinctive  AllPortsSameDT=off  OutDataTypeStr=boolean
  B-Modifier : Logic  Operator=XOR  IconShape=distinctive  AllPortsSameDT=off  OutDataTypeStr=boolean
  CE : Logic  IconShape=distinctive  AllPortsSameDT=off  OutDataTypeStr=boolean
  CI&&A^B : Logic  IconShape=distinctive  AllPortsSameDT=off  OutDataTypeStr=boolean
  CO|| : Logic  Operator=OR  IconShape=distinctive  AllPortsSameDT=off  OutDataTypeStr=boolean
  Mux : Mux  Inputs=6
  SUM : Logic  Operator=XOR  IconShape=distinctive  AllPortsSameDT=off  OutDataTypeStr=boolean
  Carry Out : Outport
  = Currently : Outport  Port=2
  A >B Next : Outport  Port=3
  Bus : Outport  Port=4
  wires:
  B/1 -> B-Modifier/1
  Subtract/1 -> B-Modifier/2
  CI&&A^B/1 -> CO||/1
  A&&B/1 -> Mux/2, CO||/2  "AND"
  CO||/1 -> Carry Out/1
  B-Modifier/1 -> A&&B/2, !B/1, A||B/2, A^B/2  "B_M"
  Carry In/1 -> CI&&A^B/2, SUM/2
  SUM/1 -> Mux/1  "Sum"
  A^B/1 -> Mux/4, CI&&A^B/1, 3AND/3, !A^B/1, SUM/1  "XOR"
  A>B Prev/1 -> ALN/1
  ALN/1 -> A >B Next/1
  !A^B/1 -> CE/2
  CE/1 -> = Currently/1
  3AND/1 -> ALN/2
  A/1 -> !A/1, A||B/1, A&&B/1, A^B/1, 3AND/2
  = So far/1 -> CE/1, 3AND/1
  A||B/1 -> Mux/3  "OR"
  Mux/1 -> Bus/1
  !A/1 -> Mux/5  "!A"
  !B/1 -> Mux/6  "!B"

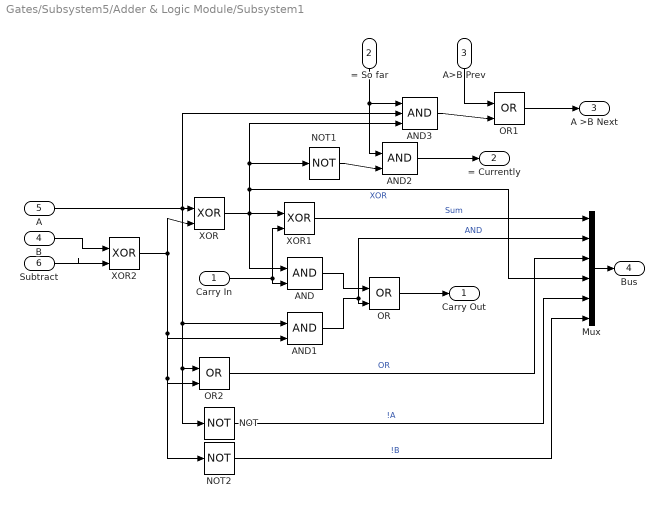
== system Gates/Subsystem5/Adder & Logic Module/Subsystem1 ==
  Carry In : Inport
  = So far : Inport  Port=2
  A>B Prev : Inport  Port=3
  B : Inport  Port=4
  A : Inport  Port=5
  Subtract : Inport  Port=6
  AND : Logic  IconShape=distinctive  AllPortsSameDT=off  OutDataTypeStr=boolean
  AND1 : Logic  IconShape=distinctive  AllPortsSameDT=off  OutDataTypeStr=boolean
  AND2 : Logic  IconShape=distinctive  AllPortsSameDT=off  OutDataTypeStr=boolean
  AND3 : Logic  Inputs=3  IconShape=distinctive  AllPortsSameDT=off  OutDataTypeStr=boolean
  Mux : Mux  Inputs=6
  NOT : Logic  Operator=NOT  IconShape=distinctive  AllPortsSameDT=off  OutDataTypeStr=boolean
  NOT1 : Logic  Operator=NOT  IconShape=distinctive  AllPortsSameDT=off  OutDataTypeStr=boolean
  NOT2 : Logic  Operator=NOT  IconShape=distinctive  AllPortsSameDT=off  OutDataTypeStr=boolean
  OR : Logic  Operator=OR  IconShape=distinctive  AllPortsSameDT=off  OutDataTypeStr=boolean
  OR1 : Logic  Operator=OR  IconShape=distinctive  AllPortsSameDT=off  OutDataTypeStr=boolean
  OR2 : Logic  Operator=OR  IconShape=distinctive  AllPortsSameDT=off  OutDataTypeStr=boolean
  XOR : Logic  Operator=XOR  IconShape=distinctive  AllPortsSameDT=off  OutDataTypeStr=boolean
  XOR1 : Logic  Operator=XOR  IconShape=distinctive  AllPortsSameDT=off  OutDataTypeStr=boolean
  XOR2 : Logic  Operator=XOR  IconShape=distinctive  AllPortsSameDT=off  OutDataTypeStr=boolean
  Carry Out : Outport
  = Currently : Outport  Port=2
  A >B Next : Outport  Port=3
  Bus : Outport  Port=4
  wires:
  B/1 -> XOR2/1
  Subtract/1 -> XOR2/2
  AND/1 -> OR/1
  AND1/1 -> Mux/2, OR/2  "AND"
  OR/1 -> Carry Out/1
  XOR2/1 -> AND1/2, NOT2/1, OR2/2, XOR/2
  Carry In/1 -> XOR1/2, AND/2
  XOR1/1 -> Mux/1  "Sum"
  XOR/1 -> Mux/4, AND3/3, NOT1/1, XOR1/1, AND/1  "XOR"
  A>B Prev/1 -> OR1/1
  OR1/1 -> A >B Next/1
  NOT1/1 -> AND2/2
  AND2/1 -> = Currently/1
  AND3/1 -> OR1/2
  A/1 -> NOT/1, OR2/1, AND1/1, XOR/1, AND3/2
  = So far/1 -> AND2/1, AND3/1
  OR2/1 -> Mux/3  "OR"
  Mux/1 -> Bus/1
  NOT/1 -> Mux/5  "!A"
  NOT2/1 -> Mux/6  "!B"

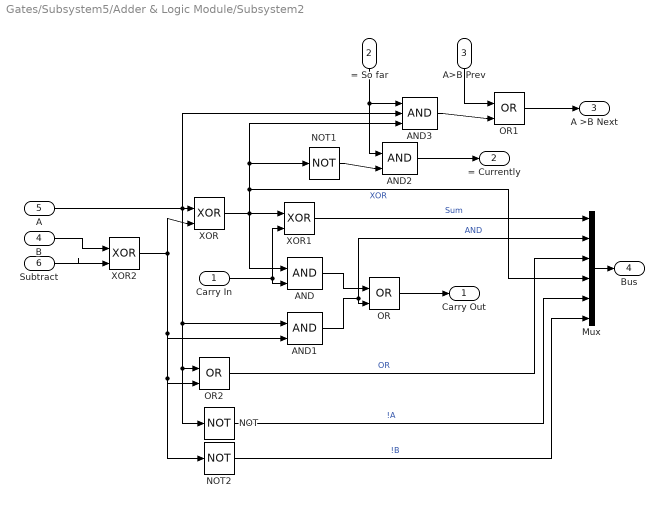
== system Gates/Subsystem5/Adder & Logic Module/Subsystem2 ==
  Carry In : Inport
  = So far : Inport  Port=2
  A>B Prev : Inport  Port=3
  B : Inport  Port=4
  A : Inport  Port=5
  Subtract : Inport  Port=6
  AND : Logic  IconShape=distinctive  AllPortsSameDT=off  OutDataTypeStr=boolean
  AND1 : Logic  IconShape=distinctive  AllPortsSameDT=off  OutDataTypeStr=boolean
  AND2 : Logic  IconShape=distinctive  AllPortsSameDT=off  OutDataTypeStr=boolean
  AND3 : Logic  Inputs=3  IconShape=distinctive  AllPortsSameDT=off  OutDataTypeStr=boolean
  Mux : Mux  Inputs=6
  NOT : Logic  Operator=NOT  IconShape=distinctive  AllPortsSameDT=off  OutDataTypeStr=boolean
  NOT1 : Logic  Operator=NOT  IconShape=distinctive  AllPortsSameDT=off  OutDataTypeStr=boolean
  NOT2 : Logic  Operator=NOT  IconShape=distinctive  AllPortsSameDT=off  OutDataTypeStr=boolean
  OR : Logic  Operator=OR  IconShape=distinctive  AllPortsSameDT=off  OutDataTypeStr=boolean
  OR1 : Logic  Operator=OR  IconShape=distinctive  AllPortsSameDT=off  OutDataTypeStr=boolean
  OR2 : Logic  Operator=OR  IconShape=distinctive  AllPortsSameDT=off  OutDataTypeStr=boolean
  XOR : Logic  Operator=XOR  IconShape=distinctive  AllPortsSameDT=off  OutDataTypeStr=boolean
  XOR1 : Logic  Operator=XOR  IconShape=distinctive  AllPortsSameDT=off  OutDataTypeStr=boolean
  XOR2 : Logic  Operator=XOR  IconShape=distinctive  AllPortsSameDT=off  OutDataTypeStr=boolean
  Carry Out : Outport
  = Currently : Outport  Port=2
  A >B Next : Outport  Port=3
  Bus : Outport  Port=4
  wires:
  B/1 -> XOR2/1
  Subtract/1 -> XOR2/2
  AND/1 -> OR/1
  AND1/1 -> Mux/2, OR/2  "AND"
  OR/1 -> Carry Out/1
  XOR2/1 -> AND1/2, NOT2/1, OR2/2, XOR/2
  Carry In/1 -> XOR1/2, AND/2
  XOR1/1 -> Mux/1  "Sum"
  XOR/1 -> Mux/4, AND3/3, NOT1/1, XOR1/1, AND/1  "XOR"
  A>B Prev/1 -> OR1/1
  OR1/1 -> A >B Next/1
  NOT1/1 -> AND2/2
  AND2/1 -> = Currently/1
  AND3/1 -> OR1/2
  A/1 -> NOT/1, OR2/1, AND1/1, XOR/1, AND3/2
  = So far/1 -> AND2/1, AND3/1
  OR2/1 -> Mux/3  "OR"
  Mux/1 -> Bus/1
  NOT/1 -> Mux/5  "!A"
  NOT2/1 -> Mux/6  "!B"

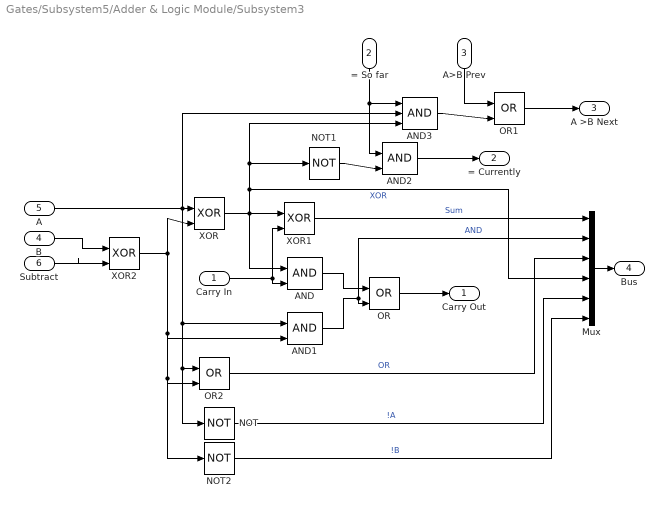
== system Gates/Subsystem5/Adder & Logic Module/Subsystem3 ==
  Carry In : Inport
  = So far : Inport  Port=2
  A>B Prev : Inport  Port=3
  B : Inport  Port=4
  A : Inport  Port=5
  Subtract : Inport  Port=6
  AND : Logic  IconShape=distinctive  AllPortsSameDT=off  OutDataTypeStr=boolean
  AND1 : Logic  IconShape=distinctive  AllPortsSameDT=off  OutDataTypeStr=boolean
  AND2 : Logic  IconShape=distinctive  AllPortsSameDT=off  OutDataTypeStr=boolean
  AND3 : Logic  Inputs=3  IconShape=distinctive  AllPortsSameDT=off  OutDataTypeStr=boolean
  Mux : Mux  Inputs=6
  NOT : Logic  Operator=NOT  IconShape=distinctive  AllPortsSameDT=off  OutDataTypeStr=boolean
  NOT1 : Logic  Operator=NOT  IconShape=distinctive  AllPortsSameDT=off  OutDataTypeStr=boolean
  NOT2 : Logic  Operator=NOT  IconShape=distinctive  AllPortsSameDT=off  OutDataTypeStr=boolean
  OR : Logic  Operator=OR  IconShape=distinctive  AllPortsSameDT=off  OutDataTypeStr=boolean
  OR1 : Logic  Operator=OR  IconShape=distinctive  AllPortsSameDT=off  OutDataTypeStr=boolean
  OR2 : Logic  Operator=OR  IconShape=distinctive  AllPortsSameDT=off  OutDataTypeStr=boolean
  XOR : Logic  Operator=XOR  IconShape=distinctive  AllPortsSameDT=off  OutDataTypeStr=boolean
  XOR1 : Logic  Operator=XOR  IconShape=distinctive  AllPortsSameDT=off  OutDataTypeStr=boolean
  XOR2 : Logic  Operator=XOR  IconShape=distinctive  AllPortsSameDT=off  OutDataTypeStr=boolean
  Carry Out : Outport
  = Currently : Outport  Port=2
  A >B Next : Outport  Port=3
  Bus : Outport  Port=4
  wires:
  B/1 -> XOR2/1
  Subtract/1 -> XOR2/2
  AND/1 -> OR/1
  AND1/1 -> Mux/2, OR/2  "AND"
  OR/1 -> Carry Out/1
  XOR2/1 -> AND1/2, NOT2/1, OR2/2, XOR/2
  Carry In/1 -> XOR1/2, AND/2
  XOR1/1 -> Mux/1  "Sum"
  XOR/1 -> Mux/4, AND3/3, NOT1/1, XOR1/1, AND/1  "XOR"
  A>B Prev/1 -> OR1/1
  OR1/1 -> A >B Next/1
  NOT1/1 -> AND2/2
  AND2/1 -> = Currently/1
  AND3/1 -> OR1/2
  A/1 -> NOT/1, OR2/1, AND1/1, XOR/1, AND3/2
  = So far/1 -> AND2/1, AND3/1
  OR2/1 -> Mux/3  "OR"
  Mux/1 -> Bus/1
  NOT/1 -> Mux/5  "!A"
  NOT2/1 -> Mux/6  "!B"

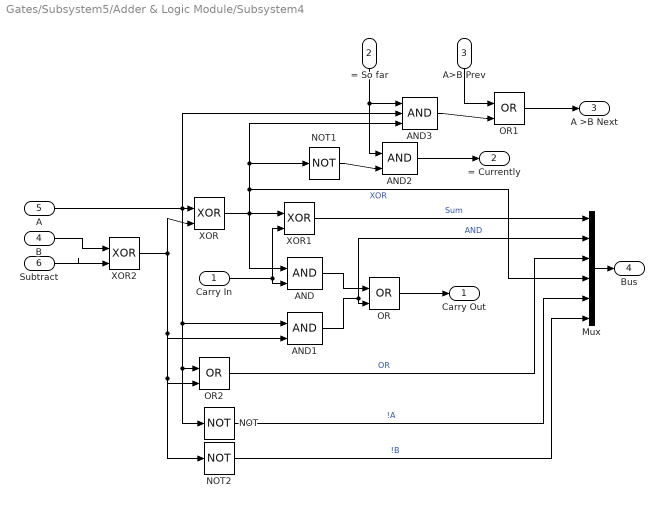
== system Gates/Subsystem5/Adder & Logic Module/Subsystem4 ==
  Carry In : Inport
  = So far : Inport  Port=2
  A>B Prev : Inport  Port=3
  B : Inport  Port=4
  A : Inport  Port=5
  Subtract : Inport  Port=6
  AND : Logic  IconShape=distinctive  AllPortsSameDT=off  OutDataTypeStr=boolean
  AND1 : Logic  IconShape=distinctive  AllPortsSameDT=off  OutDataTypeStr=boolean
  AND2 : Logic  IconShape=distinctive  AllPortsSameDT=off  OutDataTypeStr=boolean
  AND3 : Logic  Inputs=3  IconShape=distinctive  AllPortsSameDT=off  OutDataTypeStr=boolean
  Mux : Mux  Inputs=6
  NOT : Logic  Operator=NOT  IconShape=distinctive  AllPortsSameDT=off  OutDataTypeStr=boolean
  NOT1 : Logic  Operator=NOT  IconShape=distinctive  AllPortsSameDT=off  OutDataTypeStr=boolean
  NOT2 : Logic  Operator=NOT  IconShape=distinctive  AllPortsSameDT=off  OutDataTypeStr=boolean
  OR : Logic  Operator=OR  IconShape=distinctive  AllPortsSameDT=off  OutDataTypeStr=boolean
  OR1 : Logic  Operator=OR  IconShape=distinctive  AllPortsSameDT=off  OutDataTypeStr=boolean
  OR2 : Logic  Operator=OR  IconShape=distinctive  AllPortsSameDT=off  OutDataTypeStr=boolean
  XOR : Logic  Operator=XOR  IconShape=distinctive  AllPortsSameDT=off  OutDataTypeStr=boolean
  XOR1 : Logic  Operator=XOR  IconShape=distinctive  AllPortsSameDT=off  OutDataTypeStr=boolean
  XOR2 : Logic  Operator=XOR  IconShape=distinctive  AllPortsSameDT=off  OutDataTypeStr=boolean
  Carry Out : Outport
  = Currently : Outport  Port=2
  A >B Next : Outport  Port=3
  Bus : Outport  Port=4
  wires:
  B/1 -> XOR2/1
  Subtract/1 -> XOR2/2
  AND/1 -> OR/1
  AND1/1 -> Mux/2, OR/2  "AND"
  OR/1 -> Carry Out/1
  XOR2/1 -> AND1/2, NOT2/1, OR2/2, XOR/2
  Carry In/1 -> XOR1/2, AND/2
  XOR1/1 -> Mux/1  "Sum"
  XOR/1 -> Mux/4, AND3/3, NOT1/1, XOR1/1, AND/1  "XOR"
  A>B Prev/1 -> OR1/1
  OR1/1 -> A >B Next/1
  NOT1/1 -> AND2/2
  AND2/1 -> = Currently/1
  AND3/1 -> OR1/2
  A/1 -> NOT/1, OR2/1, AND1/1, XOR/1, AND3/2
  = So far/1 -> AND2/1, AND3/1
  OR2/1 -> Mux/3  "OR"
  Mux/1 -> Bus/1
  NOT/1 -> Mux/5  "!A"
  NOT2/1 -> Mux/6  "!B"

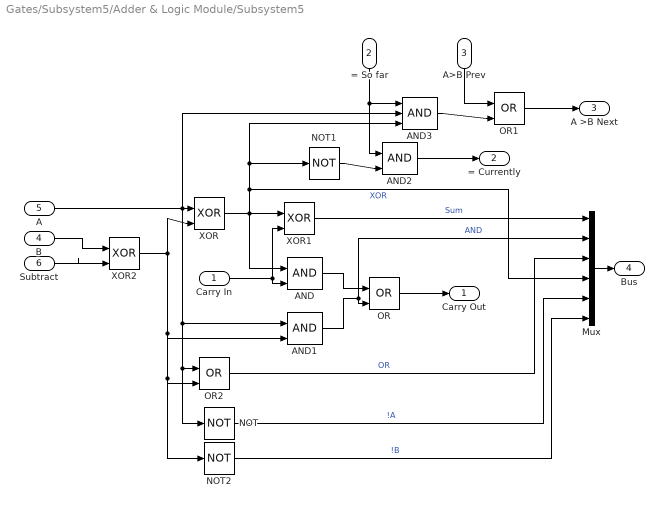
== system Gates/Subsystem5/Adder & Logic Module/Subsystem5 ==
  Carry In : Inport
  = So far : Inport  Port=2
  A>B Prev : Inport  Port=3
  B : Inport  Port=4
  A : Inport  Port=5
  Subtract : Inport  Port=6
  AND : Logic  IconShape=distinctive  AllPortsSameDT=off  OutDataTypeStr=boolean
  AND1 : Logic  IconShape=distinctive  AllPortsSameDT=off  OutDataTypeStr=boolean
  AND2 : Logic  IconShape=distinctive  AllPortsSameDT=off  OutDataTypeStr=boolean
  AND3 : Logic  Inputs=3  IconShape=distinctive  AllPortsSameDT=off  OutDataTypeStr=boolean
  Mux : Mux  Inputs=6
  NOT : Logic  Operator=NOT  IconShape=distinctive  AllPortsSameDT=off  OutDataTypeStr=boolean
  NOT1 : Logic  Operator=NOT  IconShape=distinctive  AllPortsSameDT=off  OutDataTypeStr=boolean
  NOT2 : Logic  Operator=NOT  IconShape=distinctive  AllPortsSameDT=off  OutDataTypeStr=boolean
  OR : Logic  Operator=OR  IconShape=distinctive  AllPortsSameDT=off  OutDataTypeStr=boolean
  OR1 : Logic  Operator=OR  IconShape=distinctive  AllPortsSameDT=off  OutDataTypeStr=boolean
  OR2 : Logic  Operator=OR  IconShape=distinctive  AllPortsSameDT=off  OutDataTypeStr=boolean
  XOR : Logic  Operator=XOR  IconShape=distinctive  AllPortsSameDT=off  OutDataTypeStr=boolean
  XOR1 : Logic  Operator=XOR  IconShape=distinctive  AllPortsSameDT=off  OutDataTypeStr=boolean
  XOR2 : Logic  Operator=XOR  IconShape=distinctive  AllPortsSameDT=off  OutDataTypeStr=boolean
  Carry Out : Outport
  = Currently : Outport  Port=2
  A >B Next : Outport  Port=3
  Bus : Outport  Port=4
  wires:
  B/1 -> XOR2/1
  Subtract/1 -> XOR2/2
  AND/1 -> OR/1
  AND1/1 -> Mux/2, OR/2  "AND"
  OR/1 -> Carry Out/1
  XOR2/1 -> AND1/2, NOT2/1, OR2/2, XOR/2
  Carry In/1 -> XOR1/2, AND/2
  XOR1/1 -> Mux/1  "Sum"
  XOR/1 -> Mux/4, AND3/3, NOT1/1, XOR1/1, AND/1  "XOR"
  A>B Prev/1 -> OR1/1
  OR1/1 -> A >B Next/1
  NOT1/1 -> AND2/2
  AND2/1 -> = Currently/1
  AND3/1 -> OR1/2
  A/1 -> NOT/1, OR2/1, AND1/1, XOR/1, AND3/2
  = So far/1 -> AND2/1, AND3/1
  OR2/1 -> Mux/3  "OR"
  Mux/1 -> Bus/1
  NOT/1 -> Mux/5  "!A"
  NOT2/1 -> Mux/6  "!B"
